simulink model "C_sim_matrix"  (R2015a)
settings: Solver=ode45  StartTime=0.0  StopTime=10.0  RelTol=1e-3
values from neighbouring files (symbols this model uses):
  a_1 = 1    [parameters.m]
  l_2 = 0.5    [parameters.m]
  m_l_2 = 50    [parameters.m]
settings Model: Creator=kma  LastModifiedBy=kma

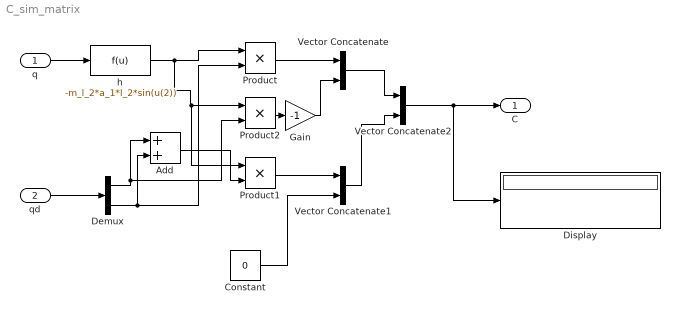
== system C_sim_matrix ==
  q : Inport  PortDimensions=2
  qd : Inport  Port=2  PortDimensions=2
  Add : Sum
  Constant : Constant  Value=0
  Demux : Demux  Outputs=2
  Display : Display
  Gain : Gain  Gain=-1
  Product : Product
  Product1 : Product
  Product2 : Product
  Vector Concatenate : Concatenate
  Vector Concatenate1 : Concatenate
  Vector Concatenate2 : Concatenate  Mode=Multidimensional array  ConcatenateDimension=2
  h : Fcn  Expr=-m_l_2*a_1*l_2*sin(u(2))
  C : Outport
  wires:
  Vector Concatenate/1 -> Vector Concatenate2/1
  Vector Concatenate1/1 -> Vector Concatenate2/2
  Vector Concatenate2/1 -> Display/1, C/1
  q/1 -> h/1
  qd/1 -> Demux/1
  Product/1 -> Vector Concatenate/1
  h/1 -> Product1/1, Product2/1, Product/1
  Demux/2 -> Add/2, Product/2
  Demux/1 -> Product2/2, Add/1
  Constant/1 -> Vector Concatenate1/2
  Product2/1 -> Gain/1
  Gain/1 -> Vector Concatenate/2
  Add/1 -> Product1/2
  Product1/1 -> Vector Concatenate1/1
